simulink model "ll1"  (Simulink 7.1)
settings: Solver=ode45  StartTime=0.0  StopTime=10.0  RelTol=1e-3
values from neighbouring files (symbols this model uses):
  Ctorque = cq(2:5:102,2:5:182)    [cq_table.m]
  R = [    R1,     0,     0,     0,     0,     0;         0,    R1,     0,     0,     0,     0;         0,     0,    R1,     0,     0,     0;         0,     0,     0,    R2,     0,     0;         0,     0,     0,     0,    R2,     0;         0,     0,     0,     0,     0,    R2]    [matrix_coeff_trafo3limb_abc.m]
undefined symbols (not defined in the file or in its folder): cut_in, cut_out, ro_air
settings Model: Creator=xc  LastModifiedBy=xc

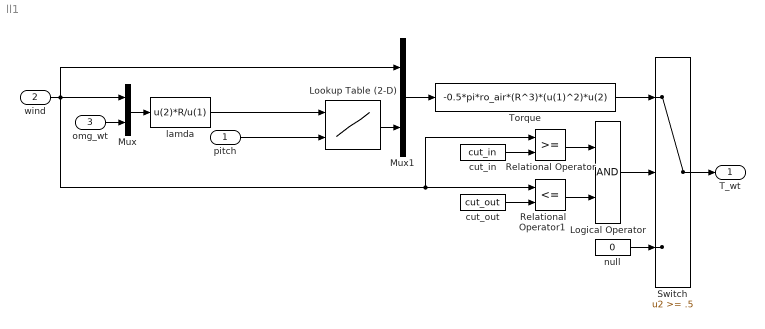
== system ll1 ==
  pitch : Inport  OutDataType=sfix(16)  OutScaling=2^0
  wind : Inport  Port=2  OutDataType=sfix(16)  OutScaling=2^0
  omg_wt : Inport  Port=3  OutDataType=sfix(16)  OutScaling=2^0
  Logical Operator : Logic
  Lookup Table (2-D) : Lookup2D  RowIndex=[0:1:20]  ColumnIndex=[-90:5:90]  Table=Ctorque  OutDataType=sfix(16)  OutScaling=2^0
  Mux : Mux  Inputs=2
  Mux1 : Mux  Inputs=2
  Relational Operator : RelationalOperator  InputSameDT=on
  Relational Operator1 : RelationalOperator  Operator=<=  InputSameDT=on
  Switch : Switch  Threshold=.5  SaturateOnIntegerOverflow=on  InputSameDT=on
  Torque : Fcn  Expr=-0.5*pi*ro_air*(R^3)*(u(1)^2)*u(2)
  cut_in : Constant  Value=cut_in  OutDataType=sfix(16)  OutScaling=2^0
  cut_out : Constant  Value=cut_out  OutDataType=sfix(16)  OutScaling=2^0
  lamda : Fcn  Expr=u(2)*R/u(1)
  null : Constant  Value=0  OutDataType=sfix(16)  OutScaling=2^0
  T_wt : Outport
  wires:
  Mux/1 -> lamda/1
  Mux1/1 -> Torque/1
  omg_wt/1 -> Mux/2
  cut_in/1 -> Relational Operator/2
  cut_out/1 -> Relational Operator1/2
  Relational Operator1/1 -> Logical Operator/2
  Relational Operator/1 -> Logical Operator/1
  Switch/1 -> T_wt/1
  Torque/1 -> Switch/1
  null/1 -> Switch/3
  Logical Operator/1 -> Switch/2
  wind/1 -> Mux/1, Relational Operator/1, Relational Operator1/1, Mux1/1
  Lookup Table (2-D)/1 -> Mux1/2
  lamda/1 -> Lookup Table (2-D)/1
  pitch/1 -> Lookup Table (2-D)/2
